simulink model "gp14_simulink"  (Simulink 8.0)
settings: Solver=ode45  StartTime=0.0  StopTime=10.0  RelTol=1e-3
undefined symbols (not defined in the file): A, B, C
libraries: dspstat3 x4, simulink x1
settings Model: Creator=Anette Andersen  LastModifiedBy=Roberto
settings OptimizationCC: InitFltsAndDblsToZero=on
settings DebuggingCC: FcnCallInpInsideContextMsg=UseLocalSettings  StrictBusMsg=Warning
settings GRTTargetCC: CombineOutputUpdateFcns=off  GRTInterface=on

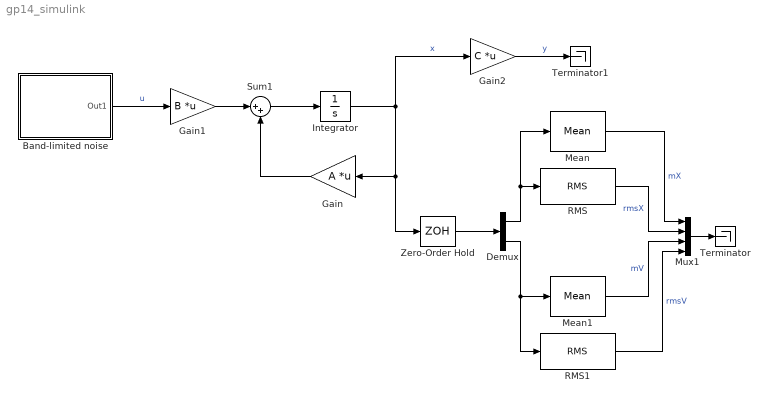
== system gp14_simulink ==
  Band-limited noise : Subsystem  mask{sigma=sqrt(0.5), beta=10, seed=171}
      mask prompts: seed "noise generator seed"
      mask help:
      | Band limited white noise with specified variance (sigma) and
      | autocorrelation function:  sigma^2 *exp(-t*beta) (t>0).
      | The seed must be diferent for different noise generators.
  Demux : Demux  Outputs=2
  Gain : Gain  Gain=A  Multiplication=Matrix(K*u)
  Gain1 : Gain  Gain=B  Multiplication=Matrix(K*u)
  Gain2 : Gain  Gain=C  Multiplication=Matrix(K*u)
  Integrator : Integrator
  Mean : dspstat3/Mean  run=on  reset_popup=None  InputProcessing=Columns as channels (frame based)  directionMode=Each column  dimension=1  treatSBRowAsCol=on  roiEnable=off  roiType=Rectangles  roiPortion=Entire ROI  roiOutput=Individual statistics for each ROI  roiFlag=off  outputDataTypeStr=Inherit: Same as accumulator  outputLastDataTypeStr=Inherit: Same as accumulator  outputMin=[]  outputMax=[]  roundingMode=Floor  overflowMode=off
  Mean1 : dspstat3/Mean  run=on  reset_popup=None  InputProcessing=Columns as channels (frame based)  directionMode=Each column  dimension=1  treatSBRowAsCol=on  roiEnable=off  roiType=Rectangles  roiPortion=Entire ROI  roiOutput=Individual statistics for each ROI  roiFlag=off  outputDataTypeStr=Inherit: Same as accumulator  outputLastDataTypeStr=Inherit: Same as accumulator  outputMin=[]  outputMax=[]  roundingMode=Floor  overflowMode=off
  Mux1 : Mux
  RMS : dspstat3/RMS  run=on  reset_popup=None  InputProcessing=Columns as channels (frame based)  directionMode=Each column  dimension=1  treatSBRowAsCol=on
  RMS1 : dspstat3/RMS  run=on  reset_popup=None  InputProcessing=Columns as channels (frame based)  directionMode=Each column  dimension=1  treatSBRowAsCol=on
  Sum1 : Sum  Inputs=|++
  Terminator : Terminator
  Terminator1 : Terminator
  Zero-Order Hold : ZeroOrderHold
  wires:
  Gain1/1 -> Sum1/1
  Sum1/1 -> Integrator/1
  Integrator/1 -> Gain/1, Zero-Order Hold/1, Gain2/1  "x"
  Gain/1 -> Sum1/2
  Demux/1 -> Mean/1, RMS/1
  Demux/2 -> RMS1/1, Mean1/1
  Zero-Order Hold/1 -> Demux/1
  Mean/1 -> Mux1/1  "mX"
  RMS/1 -> Mux1/2  "rmsX"
  Mean1/1 -> Mux1/3  "mV"
  RMS1/1 -> Mux1/4  "rmsV"
  Mux1/1 -> Terminator/1
  Band-limited noise/1(Out1) -> Gain1/1  "u"
  Gain2/1 -> Terminator1/1  "y"

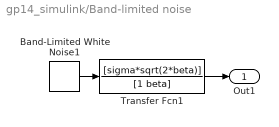
== system gp14_simulink/Band-limited noise ==
  Band-Limited White Noise1 : simulink/Sources/Band-Limited White Noise  Cov=[1]  Ts=0.15/beta  seed=seed
  Transfer Fcn1 : TransferFcn  Numerator=[sigma*sqrt(2*beta)]  Denominator=[1 beta]
  Out1 : Outport
  wires:
  Transfer Fcn1/1 -> Out1/1
  Band-Limited White Noise1/1 -> Transfer Fcn1/1
